simulink model "chap03"  (R2021a)
settings: Solver=FixedStepDiscrete  StartTime=0.0  StopTime=7.5  FixedStep=0.001  RelTol=1e-3
undefined symbols (not defined in the file): DiscIntNeverNeededParam
(part 1 of 3)
settings Model: Creator=陈天兴  LastModifiedBy=陈天兴

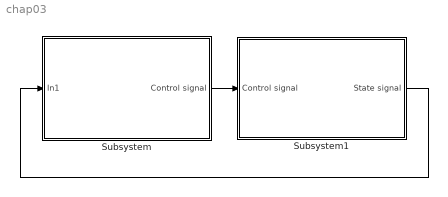
== system chap03 ==
  Subsystem : Subsystem
  Subsystem1 : Subsystem
  wires:
  Subsystem1/1(State signal) -> Subsystem/1(In1)
  Subsystem/1(Control signal) -> Subsystem1/1(Control signal)

== system chap03/Subsystem ==
  In1 : Inport
  Bus Creator : BusCreator  Inputs=6
  Bus Creator1 : BusCreator  Inputs=6
  Bus Creator2 : BusCreator  Inputs=2
  Subsystem : Subsystem
  Subsystem1 : Subsystem
  Subsystem10 : Subsystem
  Subsystem11 : Subsystem
  Subsystem12 : Subsystem
  Subsystem2 : Subsystem
  Subsystem3 : Subsystem
  Subsystem4 : Subsystem
  Subsystem5 : Subsystem
  Subsystem6 : Subsystem
  Subsystem8 : Subsystem
  Subsystem9 : Subsystem
  Control signal : Outport
  wires:
  Bus Creator2/1 -> Subsystem11/1(In19), Subsystem8/1(In19), Subsystem10/1(In19), Subsystem12/1(In19), Subsystem9/1(In19), Subsystem6/1(In19), Subsystem/1(In19), Subsystem2/1(In19), Subsystem5/1(In19), Subsystem4/1(In19), Subsystem1/1(In19), Subsystem3/1(In19)
  Subsystem5/1(u3) -> Bus Creator/3
  Subsystem3/1(u4) -> Bus Creator/4
  Subsystem1/1(u5) -> Bus Creator/5
  Subsystem/1(u1) -> Bus Creator/1
  Subsystem2/1(u2) -> Bus Creator/2
  Subsystem4/1(u6) -> Bus Creator/6
  Bus Creator/1 -> Control signal/1
  Subsystem10/1(u4) -> Bus Creator1/4
  In1/1 -> Bus Creator2/2  "state(t)"
  Bus Creator1/1 -> Bus Creator2/1  "state(tk)"
  Subsystem6/1(u1) -> Bus Creator1/1
  Subsystem9/1(u2) -> Bus Creator1/2
  Subsystem12/1(u3) -> Bus Creator1/3
  Subsystem8/1(u5) -> Bus Creator1/5
  Subsystem11/1(u6) -> Bus Creator1/6

== system chap03/Subsystem1 ==
  Control signal : Inport
  Bus Creator : BusCreator  Inputs=6
  Bus Selector : BusSelector  OutputSignals=node1.ux,node1.uy,node1.uz
  Bus Selector1 : BusSelector  OutputSignals=node2.ux,node2.uy,node2.uz
  Bus Selector2 : BusSelector  OutputSignals=node3.ux,node3.uy,node3.uz
  Bus Selector3 : BusSelector  OutputSignals=node4.ux,node4.uy,node4.uz
  Bus Selector4 : BusSelector  OutputSignals=node5.ux,node5.uy,node5.uz
  Bus Selector5 : BusSelector  OutputSignals=node6.ux,node6.uy,node6.uz
  Subsystem : Subsystem
  Subsystem1 : Subsystem
  Subsystem2 : Subsystem
  Subsystem3 : Subsystem
  Subsystem4 : Subsystem
  Subsystem5 : Subsystem
  State signal : Outport
  wires:
  Bus Creator/1 -> State signal/1
  Subsystem/1(node1) -> Bus Creator/1
  Subsystem1/1(node2) -> Bus Creator/2
  Subsystem2/1(node3) -> Bus Creator/3
  Subsystem3/1(node4) -> Bus Creator/4
  Subsystem4/1(node5) -> Bus Creator/5
  Subsystem5/1(node6) -> Bus Creator/6
  Control signal/1 -> Bus Selector2/1, Bus Selector1/1, Bus Selector/1, Bus Selector5/1, Bus Selector4/1, Bus Selector3/1
  Bus Selector/1 -> Subsystem/1(ut1x)  "<ux>"
  Bus Selector/2 -> Subsystem/2(ut1y)  "<uy>"
  Bus Selector/3 -> Subsystem/3(ut1z)  "<uz>"
  Bus Selector1/1 -> Subsystem1/1(ut2x)  "<ux>"
  Bus Selector1/2 -> Subsystem1/2(ut2y)  "<uy>"
  Bus Selector1/3 -> Subsystem1/3(ut2z)  "<uz>"
  Bus Selector2/1 -> Subsystem2/1(ut3x)  "<ux>"
  Bus Selector2/2 -> Subsystem2/2(ut3y)  "<uy>"
  Bus Selector2/3 -> Subsystem2/3(ut3z)  "<uz>"
  Bus Selector3/1 -> Subsystem3/1(ut4x)  "<ux>"
  Bus Selector3/2 -> Subsystem3/2(ut4y)  "<uy>"
  Bus Selector3/3 -> Subsystem3/3(ut4z)  "<uz>"
  Bus Selector4/1 -> Subsystem4/1(ut5x)  "<ux>"
  Bus Selector4/2 -> Subsystem4/2(ut5y)  "<uy>"
  Bus Selector4/3 -> Subsystem4/3(ut5z)  "<uz>"
  Bus Selector5/1 -> Subsystem5/1(ut6x)  "<ux>"
  Bus Selector5/2 -> Subsystem5/2(ut6y)  "<uy>"
  Bus Selector5/3 -> Subsystem5/3(ut6z)  "<uz>"

== system chap03/Subsystem/Subsystem ==
  In19 : Inport
  Bus Creator : BusCreator  Inputs=3
  Bus Selector : BusSelector  OutputSignals=state(tk).node1.xx,state(tk).node2.xx,state(tk).node3.xx,state(tk).node6.xx,state(tk).node1.vx,state(tk).node2.vx,state(tk).node3.vx,state(tk).node6.vx
  Bus Selector1 : BusSelector  OutputSignals=state(tk).node1.xy,state(tk).node2.xy,state(tk).node3.xy,state(tk).node6.xy,state(tk).node1.vy,state(tk).node2.vy,state(tk).node3.vy,state(tk).node6.vy
  Bus Selector2 : BusSelector  OutputSignals=state(tk).node1.xz,state(tk).node2.xz,state(tk).node3.xz,state(tk).node6.xz,state(tk).node1.vz,state(tk).node2.vz,state(tk).node3.vz,state(tk).node6.vz
  Subsystem1 : Subsystem
  Subsystem2 : Subsystem
  Subsystem6 : Subsystem
  u1 : Outport
  wires:
  Subsystem2/1(utx) -> Bus Creator/3  "uz"
  Subsystem6/1(utx) -> Bus Creator/1  "ux"
  Subsystem1/1(utx) -> Bus Creator/2  "uy"
  Bus Creator/1 -> u1/1  "node1"
  In19/1 -> Bus Selector2/1, Bus Selector/1, Bus Selector1/1
  Bus Selector/1 -> Subsystem6/1(xx1)  "<xx>"
  Bus Selector/2 -> Subsystem6/2(xx2)  "<xx>"
  Bus Selector/3 -> Subsystem6/3(xx3)  "<xx>"
  Bus Selector/4 -> Subsystem6/4(xx6)  "<xx>"
  Bus Selector/5 -> Subsystem6/5(vx1)  "<vx>"
  Bus Selector/6 -> Subsystem6/6(vx2)  "<vx>"
  Bus Selector/7 -> Subsystem6/7(vx3)  "<vx>"
  Bus Selector/8 -> Subsystem6/8(vx6)  "<vx>"
  Bus Selector1/1 -> Subsystem1/1(xy1)  "<xy>"
  Bus Selector1/2 -> Subsystem1/2(xy2)  "<xy>"
  Bus Selector1/3 -> Subsystem1/3(xy3)  "<xy>"
  Bus Selector1/4 -> Subsystem1/4(xy6)  "<xy>"
  Bus Selector1/5 -> Subsystem1/5(vy1)  "<vy>"
  Bus Selector1/6 -> Subsystem1/6(vy2)  "<vy>"
  Bus Selector1/7 -> Subsystem1/7(vy3)  "<vy>"
  Bus Selector1/8 -> Subsystem1/8(vy6)  "<vy>"
  Bus Selector2/1 -> Subsystem2/1(xz1)  "<xz>"
  Bus Selector2/2 -> Subsystem2/2(xx2)  "<xz>"
  Bus Selector2/3 -> Subsystem2/3(xz3)  "<xz>"
  Bus Selector2/4 -> Subsystem2/4(xz6)  "<xz>"
  Bus Selector2/5 -> Subsystem2/5(vz1)  "<vz>"
  Bus Selector2/6 -> Subsystem2/6(vz2)  "<vz>"
  Bus Selector2/7 -> Subsystem2/7(vz3)  "<vz>"
  Bus Selector2/8 -> Subsystem2/8(vz6)  "<vz>"

== system chap03/Subsystem/Subsystem1 ==
  In19 : Inport
  Bus Creator : BusCreator  Inputs=3
  Bus Selector : BusSelector  OutputSignals=state(tk).node5.xx,state(tk).node3.xx,state(tk).node4.xx,state(tk).node5.vx,state(tk).node3.vx,state(tk).node4.vx
  Bus Selector1 : BusSelector  OutputSignals=state(tk).node5.xy,state(tk).node3.xy,state(tk).node4.xy,state(tk).node5.vy,state(tk).node3.vy,state(tk).node4.vy
  Bus Selector2 : BusSelector  OutputSignals=state(tk).node5.xz,state(tk).node3.xz,state(tk).node4.xz,state(tk).node5.vz,state(tk).node3.vz,state(tk).node4.vz
  Subsystem2 : Subsystem
  Subsystem5 : Subsystem
  Subsystem6 : Subsystem
  u5 : Outport
  wires:
  Bus Creator/1 -> u5/1  "node5"
  Subsystem5/1(uty) -> Bus Creator/2  "uy"
  Subsystem6/1(utx) -> Bus Creator/1  "ux"
  Subsystem2/1(utz) -> Bus Creator/3  "uz"
  Bus Selector1/3 -> Subsystem5/3(xy4)  "<xy>"
  Bus Selector1/2 -> Subsystem5/2(xy3)  "<xy>"
  Bus Selector1/1 -> Subsystem5/1(xy5)  "<xy>"
  Bus Selector2/2 -> Subsystem2/2(xz3)  "<xz>"
  Bus Selector2/6 -> Subsystem2/6(vz4)  "<vz>"
  Bus Selector2/5 -> Subsystem2/5(vz3)  "<vz>"
  Bus Selector/4 -> Subsystem6/4(vx5)  "<vx>"
  Bus Selector1/6 -> Subsystem5/6(vy4)  "<vy>"
  Bus Selector1/4 -> Subsystem5/4(vy5)  "<vy>"
  In19/1 -> Bus Selector2/1, Bus Selector/1, Bus Selector1/1
  Bus Selector/1 -> Subsystem6/1(xx5)  "<xx>"
  Bus Selector/2 -> Subsystem6/2(xx3)  "<xx>"
  Bus Selector1/5 -> Subsystem5/5(vy3)  "<vy>"
  Bus Selector/6 -> Subsystem6/6(vx4)  "<vx>"
  Bus Selector/5 -> Subsystem6/5(vx3)  "<vx>"
  Bus Selector/3 -> Subsystem6/3(xx4)  "<xx>"
  Bus Selector2/1 -> Subsystem2/1(xz5)  "<xz>"
  Bus Selector2/3 -> Subsystem2/3(xz4)  "<xz>"
  Bus Selector2/4 -> Subsystem2/4(vz5)  "<vz>"

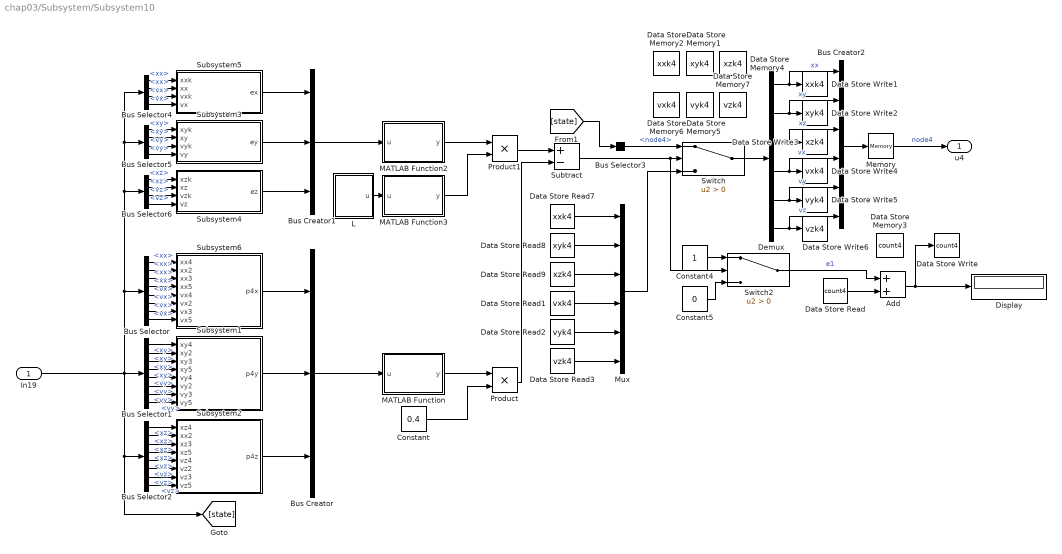
== system chap03/Subsystem/Subsystem10 ==
  In19 : Inport
  Add : Sum
  Bus Creator : BusCreator  Inputs=3
  Bus Creator1 : BusCreator  Inputs=3
  Bus Creator2 : BusCreator  Inputs=6
  Bus Selector : BusSelector  OutputSignals=state(tk).node4.xx,state(tk).node2.xx,state(tk).node3.xx,state(tk).node5.xx,state(tk).node4.vx,state(tk).node2.vx,state(tk).node3.vx,state(tk).node5.vx
  Bus Selector1 : BusSelector  OutputSignals=state(tk).node4.xy,state(tk).node2.xy,state(tk).node3.xy,state(tk).node5.xy,state(tk).node4.vy,state(tk).node2.vy,state(tk).node3.vy,state(tk).node5.vy
  Bus Selector2 : BusSelector  OutputSignals=state(tk).node4.xz,state(tk).node2.xz,state(tk).node3.xz,state(tk).node5.xz,state(tk).node4.vz,state(tk).node2.vz,state(tk).node3.vz,state(tk).node5.vz
  Bus Selector3 : BusSelector  OutputSignals=state(t).node4
  Bus Selector4 : BusSelector  OutputSignals=state(tk).node4.xx,state(t).node4.xx,state(tk).node4.vx,state(t).node4.vx
  Bus Selector5 : BusSelector  OutputSignals=state(tk).node4.xy,state(t).node4.xy,state(tk).node4.vy,state(t).node4.vy
  Bus Selector6 : BusSelector  OutputSignals=state(tk).node4.xz,state(t).node4.xz,state(tk).node4.vz,state(t).node4.vz
  Constant : Constant  Value=0.4
  Constant4 : Constant
  Constant5 : Constant  Value=0
  Data Store Memory1 : DataStoreMemory  DataStoreName=xyk4  ReadBeforeWriteMsg=warning  WriteAfterWriteMsg=warning  WriteAfterReadMsg=warning  ShowAdditionalParam=off
  Data Store Memory2 : DataStoreMemory  DataStoreName=xxk4  ReadBeforeWriteMsg=warning  WriteAfterWriteMsg=warning  WriteAfterReadMsg=warning  ShowAdditionalParam=off
  Data Store Memory3 : DataStoreMemory  DataStoreName=count4  ReadBeforeWriteMsg=warning  WriteAfterWriteMsg=warning  WriteAfterReadMsg=warning  ShowAdditionalParam=off
  Data Store Memory4 : DataStoreMemory  DataStoreName=xzk4  ReadBeforeWriteMsg=warning  WriteAfterWriteMsg=warning  WriteAfterReadMsg=warning  ShowAdditionalParam=off
  Data Store Memory5 : DataStoreMemory  DataStoreName=vyk4  ReadBeforeWriteMsg=warning  WriteAfterWriteMsg=warning  WriteAfterReadMsg=warning  ShowAdditionalParam=off
  Data Store Memory6 : DataStoreMemory  DataStoreName=vxk4  ReadBeforeWriteMsg=warning  WriteAfterWriteMsg=warning  WriteAfterReadMsg=warning  ShowAdditionalParam=off
  Data Store Memory7 : DataStoreMemory  DataStoreName=vzk4  ReadBeforeWriteMsg=warning  WriteAfterWriteMsg=warning  WriteAfterReadMsg=warning  ShowAdditionalParam=off
  Data Store Read : DataStoreRead  DataStoreName=count4  IndexOptions=Index vector (dialog)  Indices=1  OutputSizes=1
  Data Store Read1 : DataStoreRead  DataStoreName=vxk4  IndexOptions=Index vector (dialog)  Indices=1  OutputSizes=1
  Data Store Read2 : DataStoreRead  DataStoreName=vyk4  IndexOptions=Index vector (dialog)  Indices=1  OutputSizes=1
  Data Store Read3 : DataStoreRead  DataStoreName=vzk4  IndexOptions=Index vector (dialog)  Indices=1  OutputSizes=1
  Data Store Read7 : DataStoreRead  DataStoreName=xxk4  IndexOptions=Index vector (dialog)  Indices=1  OutputSizes=1
  Data Store Read8 : DataStoreRead  DataStoreName=xyk4  IndexOptions=Index vector (dialog)  Indices=1  OutputSizes=1
  Data Store Read9 : DataStoreRead  DataStoreName=xzk4  IndexOptions=Index vector (dialog)  Indices=1  OutputSizes=1
  Data Store Write : DataStoreWrite  DataStoreName=count4  IndexOptions=Index vector (dialog)  Indices=1  OutputSizes=1
  Data Store Write1 : DataStoreWrite  DataStoreName=xxk4  IndexOptions=Index vector (dialog)  Indices=1  OutputSizes=1
  Data Store Write2 : DataStoreWrite  DataStoreName=xyk4  IndexOptions=Index vector (dialog)  Indices=1  OutputSizes=1
  Data Store Write3 : DataStoreWrite  DataStoreName=xzk4  IndexOptions=Index vector (dialog)  Indices=1  OutputSizes=1
  Data Store Write4 : DataStoreWrite  DataStoreName=vxk4  IndexOptions=Index vector (dialog)  Indices=1  OutputSizes=1
  Data Store Write5 : DataStoreWrite  DataStoreName=vyk4  IndexOptions=Index vector (dialog)  Indices=1  OutputSizes=1
  Data Store Write6 : DataStoreWrite  DataStoreName=vzk4  IndexOptions=Index vector (dialog)  Indices=1  OutputSizes=1
  Demux : Demux  Outputs=6
  Display : Display
  L : Subsystem
  MATLAB Function : MATLAB Function  TreatAsAtomicUnit=on
  MATLAB Function2 : MATLAB Function  TreatAsAtomicUnit=on
  MATLAB Function3 : MATLAB Function  TreatAsAtomicUnit=on
  Memory : Memory
  Mux : Mux  Inputs=6
  Product : Product
  Product1 : Product
  Subsystem1 : Subsystem
  Subsystem2 : Subsystem
  Subsystem3 : Subsystem
  Subsystem4 : Subsystem
  Subsystem5 : Subsystem
  Subsystem6 : Subsystem
  Subtract : Sum  Inputs=+-
  Switch : Switch  Criteria=u2 > Threshold
  Switch2 : Switch  Criteria=u2 > Threshold
  u4 : Outport
  wires:
  Subsystem2/1(p4z) -> Bus Creator/3
  Subsystem6/1(p4x) -> Bus Creator/1
  Subsystem1/1(p4y) -> Bus Creator/2
  Bus Selector/1 -> Subsystem6/1(xx4)  "<xx>"
  Bus Selector/2 -> Subsystem6/2(xx2)  "<xx>"
  Bus Selector/3 -> Subsystem6/3(xx3)  "<xx>"
  Bus Selector/4 -> Subsystem6/4(xx5)  "<xx>"
  Bus Selector/5 -> Subsystem6/5(vx4)  "<vx>"
  Bus Selector/6 -> Subsystem6/6(vx2)  "<vx>"
  Bus Selector/7 -> Subsystem6/7(vx3)  "<vx>"
  Bus Selector/8 -> Subsystem6/8(vx5)  "<vx>"
  Bus Selector1/1 -> Subsystem1/1(xy4)  "<xy>"
  Bus Selector1/2 -> Subsystem1/2(xy2)  "<xy>"
  Bus Selector1/3 -> Subsystem1/3(xy3)  "<xy>"
  Bus Selector1/4 -> Subsystem1/4(xy5)  "<xy>"
  Bus Selector1/5 -> Subsystem1/5(vy4)  "<vy>"
  Bus Selector1/6 -> Subsystem1/6(vy2)  "<vy>"
  Bus Selector1/7 -> Subsystem1/7(vy3)  "<vy>"
  Bus Selector1/8 -> Subsystem1/8(vy5)  "<vy>"
  Bus Selector2/1 -> Subsystem2/1(xz4)  "<xz>"
  Bus Selector2/2 -> Subsystem2/2(xx2)  "<xz>"
  Bus Selector2/3 -> Subsystem2/3(xz3)  "<xz>"
  Bus Selector2/4 -> Subsystem2/4(xz5)  "<xz>"
  Bus Selector2/5 -> Subsystem2/5(vz4)  "<vz>"
  Bus Selector2/6 -> Subsystem2/6(vz2)  "<vz>"
  Bus Selector2/7 -> Subsystem2/7(vz3)  "<vz>"
  Bus Selector2/8 -> Subsystem2/8(vz5)  "<vz>"
  Data Store Read3/1 -> Mux/6
  Switch/1 -> Demux/1
  Demux/2 -> Bus Creator2/2, Data Store Write2/1  "xy"
  Bus Selector3/1 -> Switch/1  "<node4>"
  Demux/1 -> Bus Creator2/1, Data Store Write1/1  "xx"
  Switch2/1 -> Add/1  "e1"
  Demux/6 -> Bus Creator2/6, Data Store Write6/1  "vz"
  Demux/3 -> Bus Creator2/3, Data Store Write3/1  "xz"
  Data Store Read7/1 -> Mux/1
  Constant4/1 -> Switch2/1
  Mux/1 -> Switch/3
  Data Store Read9/1 -> Mux/3
  Add/1 -> Data Store Write/1, Display/1
  Demux/4 -> Bus Creator2/4, Data Store Write4/1  "vx"
  Bus Creator2/1 -> Memory/1
  Data Store Read2/1 -> Mux/5
  Data Store Read1/1 -> Mux/4
  Product/1 -> Subtract/2
  Data Store Read8/1 -> Mux/2
  [state] -> Bus Selector3/1
  MATLAB Function3/1(y) -> Product1/2
  Bus Creator1/1 -> MATLAB Function2/1(u)
  Constant5/1 -> Switch2/3
  Constant/1 -> Product/2
  MATLAB Function2/1(y) -> Product1/1
  Subsystem4/1(ez) -> Bus Creator1/3
  Subsystem5/1(ex) -> Bus Creator1/1
  Subsystem3/1(ey) -> Bus Creator1/2
  Demux/5 -> Bus Creator2/5, Data Store Write5/1  "vy"
  Product1/1 -> Subtract/1
  Data Store Read/1 -> Add/2
  MATLAB Function/1(y) -> Product/1
  Bus Creator/1 -> MATLAB Function/1(u)
  Bus Selector5/3 -> Subsystem3/3(vyk)  "<vy>"
  In19/1 -> [state], Bus Selector2/1, Bus Selector1/1, Bus Selector/1, Bus Selector6/1, Bus Selector5/1, Bus Selector4/1
  Bus Selector5/2 -> Subsystem3/2(xy)  "<xy>"
  Bus Selector5/4 -> Subsystem3/4(vy)  "<vy>"
  Bus Selector5/1 -> Subsystem3/1(xyk)  "<xy>"
  Bus Selector6/2 -> Subsystem4/2(xz)  "<xz>"
  Bus Selector6/3 -> Subsystem4/3(vzk)  "<vz>"
  Bus Selector6/4 -> Subsystem4/4(vz)  "<vz>"
  Bus Selector6/1 -> Subsystem4/1(xzk)  "<xz>"
  Memory/1 -> u4/1  "node4"
  Bus Selector4/1 -> Subsystem5/1(xxk)  "<xx>"
  Bus Selector4/2 -> Subsystem5/2(xx)  "<xx>"
  Bus Selector4/3 -> Subsystem5/3(vxk)  "<vx>"
  Bus Selector4/4 -> Subsystem5/4(vx)  "<vx>"
  Subtract/1 -> Switch/2, Switch2/2
  L/1(u) -> MATLAB Function3/1(u)

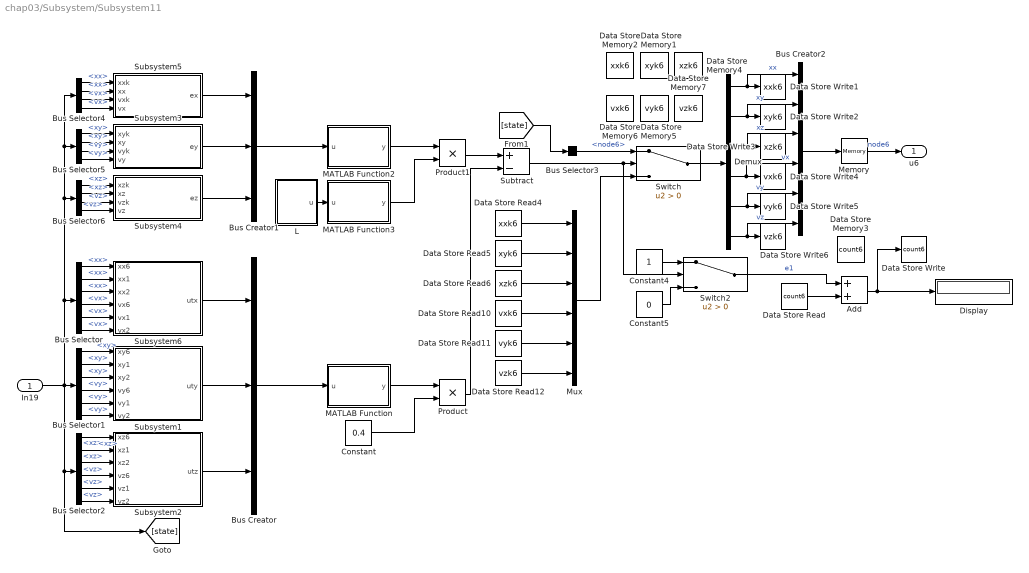
== system chap03/Subsystem/Subsystem11 ==
  In19 : Inport
  Add : Sum
  Bus Creator : BusCreator  Inputs=3
  Bus Creator1 : BusCreator  Inputs=3
  Bus Creator2 : BusCreator  Inputs=6
  Bus Selector : BusSelector  OutputSignals=state(tk).node6.xx,state(tk).node1.xx,state(tk).node2.xx,state(tk).node6.vx,state(tk).node1.vx,state(tk).node2.vx
  Bus Selector1 : BusSelector  OutputSignals=state(tk).node6.xy,state(tk).node1.xy,state(tk).node2.xy,state(tk).node6.vy,state(tk).node1.vy,state(tk).node2.vy
  Bus Selector2 : BusSelector  OutputSignals=state(tk).node6.xz,state(tk).node1.xz,state(tk).node2.xz,state(tk).node6.vz,state(tk).node1.vz,state(tk).node2.vz
  Bus Selector3 : BusSelector  OutputSignals=state(t).node6
  Bus Selector4 : BusSelector  OutputSignals=state(tk).node6.xx,state(t).node6.xx,state(tk).node6.vx,state(t).node6.vx
  Bus Selector5 : BusSelector  OutputSignals=state(tk).node6.xy,state(t).node6.xy,state(tk).node6.vy,state(t).node6.vy
  Bus Selector6 : BusSelector  OutputSignals=state(tk).node6.xz,state(t).node6.xz,state(tk).node6.vz,state(t).node6.vz
  Constant : Constant  Value=0.4
  Constant4 : Constant
  Constant5 : Constant  Value=0
  Data Store Memory1 : DataStoreMemory  DataStoreName=xyk6  ReadBeforeWriteMsg=warning  WriteAfterWriteMsg=warning  WriteAfterReadMsg=warning  ShowAdditionalParam=off
  Data Store Memory2 : DataStoreMemory  DataStoreName=xxk6  ReadBeforeWriteMsg=warning  WriteAfterWriteMsg=warning  WriteAfterReadMsg=warning  ShowAdditionalParam=off
  Data Store Memory3 : DataStoreMemory  DataStoreName=count6  ReadBeforeWriteMsg=warning  WriteAfterWriteMsg=warning  WriteAfterReadMsg=warning  ShowAdditionalParam=off
  Data Store Memory4 : DataStoreMemory  DataStoreName=xzk6  ReadBeforeWriteMsg=warning  WriteAfterWriteMsg=warning  WriteAfterReadMsg=warning  ShowAdditionalParam=off
  Data Store Memory5 : DataStoreMemory  DataStoreName=vyk6  ReadBeforeWriteMsg=warning  WriteAfterWriteMsg=warning  WriteAfterReadMsg=warning  ShowAdditionalParam=off
  Data Store Memory6 : DataStoreMemory  DataStoreName=vxk6  ReadBeforeWriteMsg=warning  WriteAfterWriteMsg=warning  WriteAfterReadMsg=warning  ShowAdditionalParam=off
  Data Store Memory7 : DataStoreMemory  DataStoreName=vzk6  ReadBeforeWriteMsg=warning  WriteAfterWriteMsg=warning  WriteAfterReadMsg=warning  ShowAdditionalParam=off
  Data Store Read : DataStoreRead  DataStoreName=count6  IndexOptions=Index vector (dialog)  Indices=1  OutputSizes=1
  Data Store Read10 : DataStoreRead  DataStoreName=vxk6  IndexOptions=Index vector (dialog)  Indices=1  OutputSizes=1
  Data Store Read11 : DataStoreRead  DataStoreName=vyk6  IndexOptions=Index vector (dialog)  Indices=1  OutputSizes=1
  Data Store Read12 : DataStoreRead  DataStoreName=vzk6  IndexOptions=Index vector (dialog)  Indices=1  OutputSizes=1
  Data Store Read4 : DataStoreRead  DataStoreName=xxk6  IndexOptions=Index vector (dialog)  Indices=1  OutputSizes=1
  Data Store Read5 : DataStoreRead  DataStoreName=xyk6  IndexOptions=Index vector (dialog)  Indices=1  OutputSizes=1
  Data Store Read6 : DataStoreRead  DataStoreName=xzk6  IndexOptions=Index vector (dialog)  Indices=1  OutputSizes=1
  Data Store Write : DataStoreWrite  DataStoreName=count6  IndexOptions=Index vector (dialog)  Indices=1  OutputSizes=1
  Data Store Write1 : DataStoreWrite  DataStoreName=xxk6  IndexOptions=Index vector (dialog)  Indices=1  OutputSizes=1
  Data Store Write2 : DataStoreWrite  DataStoreName=xyk6  IndexOptions=Index vector (dialog)  Indices=1  OutputSizes=1
  Data Store Write3 : DataStoreWrite  DataStoreName=xzk6  IndexOptions=Index vector (dialog)  Indices=1  OutputSizes=1
  Data Store Write4 : DataStoreWrite  DataStoreName=vxk6  IndexOptions=Index vector (dialog)  Indices=1  OutputSizes=1
  Data Store Write5 : DataStoreWrite  DataStoreName=vyk6  IndexOptions=Index vector (dialog)  Indices=1  OutputSizes=1
  Data Store Write6 : DataStoreWrite  DataStoreName=vzk6  IndexOptions=Index vector (dialog)  Indices=1  OutputSizes=1
  Demux : Demux  Outputs=6
  Display : Display
  L : Subsystem
  MATLAB Function : MATLAB Function  TreatAsAtomicUnit=on
  MATLAB Function2 : MATLAB Function  TreatAsAtomicUnit=on
  MATLAB Function3 : MATLAB Function  TreatAsAtomicUnit=on
  Memory : Memory
  Mux : Mux  Inputs=6
  Product : Product
  Product1 : Product
  Subsystem1 : Subsystem
  Subsystem2 : Subsystem
  Subsystem3 : Subsystem
  Subsystem4 : Subsystem
  Subsystem5 : Subsystem
  Subsystem6 : Subsystem
  Subtract : Sum  Inputs=+-
  Switch : Switch  Criteria=u2 > Threshold
  Switch2 : Switch  Criteria=u2 > Threshold
  u6 : Outport
  wires:
  Bus Selector2/6 -> Subsystem2/6(vz2)  "<vz>"
  Bus Selector2/5 -> Subsystem2/5(vz1)  "<vz>"
  Bus Selector2/4 -> Subsystem2/4(vz6)  "<vz>"
  Bus Selector2/3 -> Subsystem2/3(xz2)  "<xz>"
  Bus Selector2/1 -> Subsystem2/1(xz6)  "<xz>"
  Bus Selector2/2 -> Subsystem2/2(xz1)  "<xz>"
  Bus Selector1/6 -> Subsystem1/6(vy2)  "<vy>"
  Bus Selector1/5 -> Subsystem1/5(vy1)  "<vy>"
  Bus Selector1/4 -> Subsystem1/4(vy6)  "<vy>"
  Bus Selector1/3 -> Subsystem1/3(xy2)  "<xy>"
  Bus Selector1/2 -> Subsystem1/2(xy1)  "<xy>"
  Bus Selector1/1 -> Subsystem1/1(xy6)  "<xy>"
  Bus Selector/6 -> Subsystem6/6(vx2)  "<vx>"
  Bus Selector/5 -> Subsystem6/5(vx1)  "<vx>"
  Bus Selector/4 -> Subsystem6/4(vx6)  "<vx>"
  Bus Selector/3 -> Subsystem6/3(xx2)  "<xx>"
  Bus Selector/2 -> Subsystem6/2(xx1)  "<xx>"
  Bus Selector/1 -> Subsystem6/1(xx6)  "<xx>"
  Subsystem1/1(uty) -> Bus Creator/2
  Subsystem6/1(utx) -> Bus Creator/1
  Subsystem2/1(utz) -> Bus Creator/3
  Data Store Read/1 -> Add/2
  Subsystem3/1(ey) -> Bus Creator1/2
  Demux/4 -> Bus Creator2/4, Data Store Write4/1  "vx"
  MATLAB Function/1(y) -> Product/1
  Bus Creator/1 -> MATLAB Function/1(u)
  Product1/1 -> Subtract/1
  Data Store Read4/1 -> Mux/1
  Demux/1 -> Bus Creator2/1, Data Store Write1/1  "xx"
  Add/1 -> Data Store Write/1, Display/1
  Demux/6 -> Bus Creator2/6, Data Store Write6/1  "vz"
  Subsystem5/1(ex) -> Bus Creator1/1
  Data Store Read5/1 -> Mux/2
  Demux/5 -> Bus Creator2/5, Data Store Write5/1  "vy"
  Data Store Read11/1 -> Mux/5
  Demux/3 -> Bus Creator2/3, Data Store Write3/1  "xz"
  Subsystem4/1(ez) -> Bus Creator1/3
  Bus Creator1/1 -> MATLAB Function2/1(u)
  Data Store Read6/1 -> Mux/3
  MATLAB Function2/1(y) -> Product1/1
  Constant4/1 -> Switch2/1
  Mux/1 -> Switch/3
  Switch/1 -> Demux/1
  Constant/1 -> Product/2
  Constant5/1 -> Switch2/3
  MATLAB Function3/1(y) -> Product1/2
  Data Store Read10/1 -> Mux/4
  Data Store Read12/1 -> Mux/6
  Switch2/1 -> Add/1  "e1"
  Demux/2 -> Bus Creator2/2, Data Store Write2/1  "xy"
  Product/1 -> Subtract/2
  Memory/1 -> u6/1  "node6"
  Bus Selector3/1 -> Switch/1  "<node6>"
  [state] -> Bus Selector3/1
  Bus Selector4/4 -> Subsystem5/4(vx)  "<vx>"
  Bus Selector5/3 -> Subsystem3/3(vyk)  "<vy>"
  Bus Selector5/2 -> Subsystem3/2(xy)  "<xy>"
  Bus Selector4/1 -> Subsystem5/1(xxk)  "<xx>"
  Bus Selector5/4 -> Subsystem3/4(vy)  "<vy>"
  Bus Selector5/1 -> Subsystem3/1(xyk)  "<xy>"
  In19/1 -> Bus Selector5/1, Bus Selector4/1, Bus Selector6/1, Bus Selector/1, Bus Selector1/1, [state], Bus Selector2/1
  Bus Selector4/3 -> Subsystem5/3(vxk)  "<vx>"
  Bus Selector6/2 -> Subsystem4/2(xz)  "<xz>"
  Bus Selector6/3 -> Subsystem4/3(vzk)  "<vz>"
  Bus Selector4/2 -> Subsystem5/2(xx)  "<xx>"
  Bus Selector6/4 -> Subsystem4/4(vz)  "<vz>"
  Bus Selector6/1 -> Subsystem4/1(xzk)  "<xz>"
  Bus Creator2/1 -> Memory/1
  Subtract/1 -> Switch/2, Switch2/2
  L/1(u) -> MATLAB Function3/1(u)

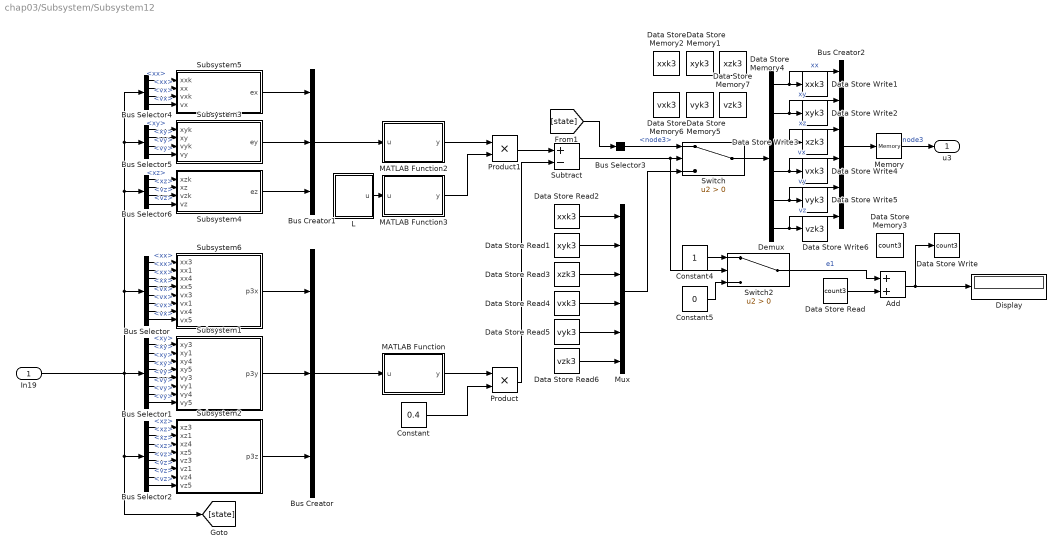
== system chap03/Subsystem/Subsystem12 ==
  In19 : Inport
  Add : Sum
  Bus Creator : BusCreator  Inputs=3
  Bus Creator1 : BusCreator  Inputs=3
  Bus Creator2 : BusCreator  Inputs=6
  Bus Selector : BusSelector  OutputSignals=state(tk).node3.xx,state(tk).node1.xx,state(tk).node4.xx,state(tk).node5.xx,state(tk).node3.vx,state(tk).node1.vx,state(tk).node4.vx,state(tk).node5.vx
  Bus Selector1 : BusSelector  OutputSignals=state(tk).node3.xy,state(tk).node1.xy,state(tk).node4.xy,state(tk).node5.xy,state(tk).node3.vy,state(tk).node1.vy,state(tk).node4.vy,state(tk).node5.vy
  Bus Selector2 : BusSelector  OutputSignals=state(tk).node3.xz,state(tk).node1.xz,state(tk).node4.xz,state(tk).node5.xz,state(tk).node3.vz,state(tk).node1.vz,state(tk).node4.vz,state(tk).node5.vz
  Bus Selector3 : BusSelector  OutputSignals=state(t).node3
  Bus Selector4 : BusSelector  OutputSignals=state(tk).node3.xx,state(t).node3.xx,state(tk).node3.vx,state(t).node3.vx
  Bus Selector5 : BusSelector  OutputSignals=state(tk).node3.xy,state(t).node3.xy,state(tk).node3.vy,state(t).node3.vy
  Bus Selector6 : BusSelector  OutputSignals=state(tk).node3.xz,state(t).node3.xz,state(tk).node3.vz,state(t).node3.vz
  Constant : Constant  Value=0.4
  Constant4 : Constant
  Constant5 : Constant  Value=0
  Data Store Memory1 : DataStoreMemory  DataStoreName=xyk3  ReadBeforeWriteMsg=warning  WriteAfterWriteMsg=warning  WriteAfterReadMsg=warning  ShowAdditionalParam=off
  Data Store Memory2 : DataStoreMemory  DataStoreName=xxk3  ReadBeforeWriteMsg=warning  WriteAfterWriteMsg=warning  WriteAfterReadMsg=warning  ShowAdditionalParam=off
  Data Store Memory3 : DataStoreMemory  DataStoreName=count3  ReadBeforeWriteMsg=warning  WriteAfterWriteMsg=warning  WriteAfterReadMsg=warning  ShowAdditionalParam=off
  Data Store Memory4 : DataStoreMemory  DataStoreName=xzk3  ReadBeforeWriteMsg=warning  WriteAfterWriteMsg=warning  WriteAfterReadMsg=warning  ShowAdditionalParam=off
  Data Store Memory5 : DataStoreMemory  DataStoreName=vyk3  ReadBeforeWriteMsg=warning  WriteAfterWriteMsg=warning  WriteAfterReadMsg=warning  ShowAdditionalParam=off
  Data Store Memory6 : DataStoreMemory  DataStoreName=vxk3  ReadBeforeWriteMsg=warning  WriteAfterWriteMsg=warning  WriteAfterReadMsg=warning  ShowAdditionalParam=off
  Data Store Memory7 : DataStoreMemory  DataStoreName=vzk3  ReadBeforeWriteMsg=warning  WriteAfterWriteMsg=warning  WriteAfterReadMsg=warning  ShowAdditionalParam=off
  Data Store Read : DataStoreRead  DataStoreName=count3  IndexOptions=Index vector (dialog)  Indices=1  OutputSizes=1
  Data Store Read1 : DataStoreRead  DataStoreName=xyk3  IndexOptions=Index vector (dialog)  Indices=1  OutputSizes=1
  Data Store Read2 : DataStoreRead  DataStoreName=xxk3  IndexOptions=Index vector (dialog)  Indices=1  OutputSizes=1
  Data Store Read3 : DataStoreRead  DataStoreName=xzk3  IndexOptions=Index vector (dialog)  Indices=1  OutputSizes=1
  Data Store Read4 : DataStoreRead  DataStoreName=vxk3  IndexOptions=Index vector (dialog)  Indices=1  OutputSizes=1
  Data Store Read5 : DataStoreRead  DataStoreName=vyk3  IndexOptions=Index vector (dialog)  Indices=1  OutputSizes=1
  Data Store Read6 : DataStoreRead  DataStoreName=vzk3  IndexOptions=Index vector (dialog)  Indices=1  OutputSizes=1
  Data Store Write : DataStoreWrite  DataStoreName=count3  IndexOptions=Index vector (dialog)  Indices=1  OutputSizes=1
  Data Store Write1 : DataStoreWrite  DataStoreName=xxk3  IndexOptions=Index vector (dialog)  Indices=1  OutputSizes=1
  Data Store Write2 : DataStoreWrite  DataStoreName=xyk3  IndexOptions=Index vector (dialog)  Indices=1  OutputSizes=1
  Data Store Write3 : DataStoreWrite  DataStoreName=xzk3  IndexOptions=Index vector (dialog)  Indices=1  OutputSizes=1
  Data Store Write4 : DataStoreWrite  DataStoreName=vxk3  IndexOptions=Index vector (dialog)  Indices=1  OutputSizes=1
  Data Store Write5 : DataStoreWrite  DataStoreName=vyk3  IndexOptions=Index vector (dialog)  Indices=1  OutputSizes=1
  Data Store Write6 : DataStoreWrite  DataStoreName=vzk3  IndexOptions=Index vector (dialog)  Indices=1  OutputSizes=1
  Demux : Demux  Outputs=6
  Display : Display
  L : Subsystem
  MATLAB Function : MATLAB Function  TreatAsAtomicUnit=on
  MATLAB Function2 : MATLAB Function  TreatAsAtomicUnit=on
  MATLAB Function3 : MATLAB Function  TreatAsAtomicUnit=on
  Memory : Memory
  Mux : Mux  Inputs=6
  Product : Product
  Product1 : Product
  Subsystem1 : Subsystem
  Subsystem2 : Subsystem
  Subsystem3 : Subsystem
  Subsystem4 : Subsystem
  Subsystem5 : Subsystem
  Subsystem6 : Subsystem
  Subtract : Sum  Inputs=+-
  Switch : Switch  Criteria=u2 > Threshold
  Switch2 : Switch  Criteria=u2 > Threshold
  u3 : Outport
  wires:
  Bus Selector2/8 -> Subsystem2/8(vz5)  "<vz>"
  Bus Selector2/7 -> Subsystem2/7(vz4)  "<vz>"
  Bus Selector2/6 -> Subsystem2/6(vz1)  "<vz>"
  Bus Selector2/5 -> Subsystem2/5(vz3)  "<vz>"
  Bus Selector2/4 -> Subsystem2/4(xz5)  "<xz>"
  Bus Selector2/3 -> Subsystem2/3(xz4)  "<xz>"
  Bus Selector2/2 -> Subsystem2/2(xz1)  "<xz>"
  Bus Selector2/1 -> Subsystem2/1(xz3)  "<xz>"
  Bus Selector1/8 -> Subsystem1/8(vy5)  "<vy>"
  Bus Selector1/7 -> Subsystem1/7(vy4)  "<vy>"
  Bus Selector1/6 -> Subsystem1/6(vy1)  "<vy>"
  Bus Selector1/5 -> Subsystem1/5(vy3)  "<vy>"
  Bus Selector1/4 -> Subsystem1/4(xy5)  "<xy>"
  Bus Selector1/3 -> Subsystem1/3(xy4)  "<xy>"
  Bus Selector1/2 -> Subsystem1/2(xy1)  "<xy>"
  Bus Selector1/1 -> Subsystem1/1(xy3)  "<xy>"
  Bus Selector/8 -> Subsystem6/8(vx5)  "<vx>"
  Bus Selector/7 -> Subsystem6/7(vx4)  "<vx>"
  Bus Selector/6 -> Subsystem6/6(vx1)  "<vx>"
  Bus Selector/5 -> Subsystem6/5(vx3)  "<vx>"
  Bus Selector/4 -> Subsystem6/4(xx5)  "<xx>"
  Bus Selector/3 -> Subsystem6/3(xx4)  "<xx>"
  Bus Selector/2 -> Subsystem6/2(xx1)  "<xx>"
  Bus Selector/1 -> Subsystem6/1(xx3)  "<xx>"
  Subsystem1/1(p3y) -> Bus Creator/2
  Subsystem6/1(p3x) -> Bus Creator/1
  Subsystem2/1(p3z) -> Bus Creator/3
  Data Store Read6/1 -> Mux/6
  Switch/1 -> Demux/1
  Demux/2 -> Bus Creator2/2, Data Store Write2/1  "xy"
  Bus Selector3/1 -> Switch/1  "<node3>"
  Demux/1 -> Bus Creator2/1, Data Store Write1/1  "xx"
  Switch2/1 -> Add/1  "e1"
  Demux/6 -> Bus Creator2/6, Data Store Write6/1  "vz"
  Demux/3 -> Bus Creator2/3, Data Store Write3/1  "xz"
  Data Store Read2/1 -> Mux/1
  Constant4/1 -> Switch2/1
  Mux/1 -> Switch/3
  Data Store Read3/1 -> Mux/3
  Add/1 -> Data Store Write/1, Display/1
  Demux/4 -> Bus Creator2/4, Data Store Write4/1  "vx"
  Memory/1 -> u3/1  "node3"
  Data Store Read5/1 -> Mux/5
  Data Store Read4/1 -> Mux/4
  Product/1 -> Subtract/2
  Data Store Read1/1 -> Mux/2
  [state] -> Bus Selector3/1
  MATLAB Function3/1(y) -> Product1/2
  Bus Creator1/1 -> MATLAB Function2/1(u)
  Constant5/1 -> Switch2/3
  Constant/1 -> Product/2
  MATLAB Function2/1(y) -> Product1/1
  Subsystem4/1(ez) -> Bus Creator1/3
  Subsystem5/1(ex) -> Bus Creator1/1
  Subsystem3/1(ey) -> Bus Creator1/2
  Demux/5 -> Bus Creator2/5, Data Store Write5/1  "vy"
  Product1/1 -> Subtract/1
  Data Store Read/1 -> Add/2
  MATLAB Function/1(y) -> Product/1
  Bus Creator/1 -> MATLAB Function/1(u)
  Bus Selector6/4 -> Subsystem4/4(vz)  "<vz>"
  Bus Selector6/2 -> Subsystem4/2(xz)  "<xz>"
  Bus Selector6/3 -> Subsystem4/3(vzk)  "<vz>"
  Bus Selector6/1 -> Subsystem4/1(xzk)  "<xz>"
  Bus Selector5/3 -> Subsystem3/3(vyk)  "<vy>"
  Bus Selector5/2 -> Subsystem3/2(xy)  "<xy>"
  Bus Selector5/4 -> Subsystem3/4(vy)  "<vy>"
  Bus Selector5/1 -> Subsystem3/1(xyk)  "<xy>"
  In19/1 -> [state], Bus Selector2/1, Bus Selector/1, Bus Selector6/1, Bus Selector5/1, Bus Selector4/1, Bus Selector1/1
  Bus Selector4/1 -> Subsystem5/1(xxk)  "<xx>"
  Bus Selector4/2 -> Subsystem5/2(xx)  "<xx>"
  Bus Selector4/3 -> Subsystem5/3(vxk)  "<vx>"
  Bus Selector4/4 -> Subsystem5/4(vx)  "<vx>"
  Bus Creator2/1 -> Memory/1
  Subtract/1 -> Switch2/2, Switch/2
  L/1(u) -> MATLAB Function3/1(u)

== system chap03/Subsystem/Subsystem2 ==
  In19 : Inport
  Bus Creator : BusCreator  Inputs=3
  Bus Selector : BusSelector  OutputSignals=state(tk).node2.xx,state(tk).node1.xx,state(tk).node4.xx,state(tk).node6.xx,state(tk).node2.vx,state(tk).node1.vx,state(tk).node4.vx,state(tk).node6.vx
  Bus Selector1 : BusSelector  OutputSignals=state(tk).node2.xy,state(tk).node1.xy,state(tk).node4.xy,state(tk).node6.xy,state(tk).node2.vy,state(tk).node1.vy,state(tk).node4.vy,state(tk).node6.vy
  Bus Selector2 : BusSelector  OutputSignals=state(tk).node2.xz,state(tk).node1.xz,state(tk).node4.xz,state(tk).node6.xz,state(tk).node2.vz,state(tk).node1.vz,state(tk).node4.vz,state(tk).node6.vz
  Subsystem1 : Subsystem
  Subsystem2 : Subsystem
  Subsystem6 : Subsystem
  u2 : Outport
  wires:
  Bus Creator/1 -> u2/1  "node2"
  Subsystem1/1(uty) -> Bus Creator/2  "uy"
  Subsystem6/1(utx) -> Bus Creator/1  "ux"
  Subsystem2/1(utz) -> Bus Creator/3  "uz"
  Bus Selector2/1 -> Subsystem2/1(xz2)  "<xz>"
  In19/1 -> Bus Selector2/1, Bus Selector/1, Bus Selector1/1
  Bus Selector/3 -> Subsystem6/3(xx4)  "<xx>"
  Bus Selector/5 -> Subsystem6/5(vx2)  "<vx>"
  Bus Selector/1 -> Subsystem6/1(xx2)  "<xx>"
  Bus Selector/7 -> Subsystem6/7(vx4)  "<vx>"
  Bus Selector1/2 -> Subsystem1/2(xy1)  "<xy>"
  Bus Selector2/4 -> Subsystem2/4(xz6)  "<xz>"
  Bus Selector2/6 -> Subsystem2/6(vz1)  "<vz>"
  Bus Selector1/1 -> Subsystem1/1(xy2)  "<xy>"
  Bus Selector2/7 -> Subsystem2/7(vz4)  "<vz>"
  Bus Selector2/5 -> Subsystem2/5(vz2)  "<vz>"
  Bus Selector1/6 -> Subsystem1/6(vy1)  "<vy>"
  Bus Selector/2 -> Subsystem6/2(xx1)  "<xx>"
  Bus Selector1/8 -> Subsystem1/8(vy6)  "<vy>"
  Bus Selector2/8 -> Subsystem2/8(vz6)  "<vz>"
  Bus Selector1/7 -> Subsystem1/7(vy4)  "<vy>"
  Bus Selector2/2 -> Subsystem2/2(xz1)  "<xz>"
  Bus Selector/8 -> Subsystem6/8(vx6)  "<vx>"
  Bus Selector1/3 -> Subsystem1/3(xy4)  "<xy>"
  Bus Selector/6 -> Subsystem6/6(vx1)  "<vx>"
  Bus Selector1/4 -> Subsystem1/4(xy6)  "<xy>"
  Bus Selector1/5 -> Subsystem1/5(vy2)  "<vy>"
  Bus Selector2/3 -> Subsystem2/3(xz4)  "<xz>"
  Bus Selector/4 -> Subsystem6/4(xx6)  "<xx>"

== system chap03/Subsystem/Subsystem3 ==
  In19 : Inport
  Bus Creator : BusCreator  Inputs=3
  Bus Selector : BusSelector  OutputSignals=state(tk).node4.xx,state(tk).node2.xx,state(tk).node3.xx,state(tk).node5.xx,state(tk).node4.vx,state(tk).node2.vx,state(tk).node3.vx,state(tk).node5.vx
  Bus Selector1 : BusSelector  OutputSignals=state(tk).node4.xy,state(tk).node2.xy,state(tk).node3.xy,state(tk).node5.xy,state(tk).node4.vy,state(tk).node2.vy,state(tk).node3.vy,state(tk).node5.vy
  Bus Selector2 : BusSelector  OutputSignals=state(tk).node4.xz,state(tk).node2.xz,state(tk).node3.xz,state(tk).node5.xz,state(tk).node4.vz,state(tk).node2.vz,state(tk).node3.vz,state(tk).node5.vz
  Subsystem1 : Subsystem
  Subsystem2 : Subsystem
  Subsystem6 : Subsystem
  u4 : Outport
  wires:
  Bus Creator/1 -> u4/1  "node4"
  Subsystem1/1(utx) -> Bus Creator/2  "uy"
  Subsystem6/1(utx) -> Bus Creator/1  "ux"
  Subsystem2/1(utx) -> Bus Creator/3  "uz"
  Bus Selector/2 -> Subsystem6/2(xx2)  "<xx>"
  Bus Selector1/7 -> Subsystem1/7(vy3)  "<vy>"
  Bus Selector1/4 -> Subsystem1/4(xy5)  "<xy>"
  Bus Selector2/3 -> Subsystem2/3(xz3)  "<xz>"
  Bus Selector/8 -> Subsystem6/8(vx5)  "<vx>"
  Bus Selector2/2 -> Subsystem2/2(xx2)  "<xz>"
  Bus Selector2/4 -> Subsystem2/4(xz5)  "<xz>"
  Bus Selector1/5 -> Subsystem1/5(vy4)  "<vy>"
  Bus Selector1/2 -> Subsystem1/2(xy2)  "<xy>"
  Bus Selector2/7 -> Subsystem2/7(vz3)  "<vz>"
  Bus Selector2/5 -> Subsystem2/5(vz4)  "<vz>"
  Bus Selector1/6 -> Subsystem1/6(vy2)  "<vy>"
  Bus Selector2/8 -> Subsystem2/8(vz5)  "<vz>"
  Bus Selector2/6 -> Subsystem2/6(vz2)  "<vz>"
  Bus Selector1/3 -> Subsystem1/3(xy3)  "<xy>"
  Bus Selector2/1 -> Subsystem2/1(xz4)  "<xz>"
  Bus Selector/5 -> Subsystem6/5(vx4)  "<vx>"
  Bus Selector/1 -> Subsystem6/1(xx4)  "<xx>"
  Bus Selector/3 -> Subsystem6/3(xx3)  "<xx>"
  In19/1 -> Bus Selector2/1, Bus Selector/1, Bus Selector1/1
  Bus Selector1/8 -> Subsystem1/8(vy5)  "<vy>"
  Bus Selector1/1 -> Subsystem1/1(xy4)  "<xy>"
  Bus Selector/7 -> Subsystem6/7(vx3)  "<vx>"
  Bus Selector/6 -> Subsystem6/6(vx2)  "<vx>"
  Bus Selector/4 -> Subsystem6/4(xx5)  "<xx>"

== system chap03/Subsystem/Subsystem4 ==
  In19 : Inport
  Bus Creator : BusCreator  Inputs=3
  Bus Selector : BusSelector  OutputSignals=state(tk).node6.xx,state(tk).node1.xx,state(tk).node2.xx,state(tk).node6.vx,state(tk).node1.vx,state(tk).node2.vx
  Bus Selector1 : BusSelector  OutputSignals=state(tk).node6.xy,state(tk).node1.xy,state(tk).node2.xy,state(tk).node6.vy,state(tk).node1.vy,state(tk).node2.vy
  Bus Selector2 : BusSelector  OutputSignals=state(tk).node6.xz,state(tk).node1.xz,state(tk).node2.xz,state(tk).node6.vz,state(tk).node1.vz,state(tk).node2.vz
  Subsystem1 : Subsystem
  Subsystem2 : Subsystem
  Subsystem6 : Subsystem
  u6 : Outport
  wires:
  Subsystem2/1(utz) -> Bus Creator/3  "uz"
  Subsystem6/1(utx) -> Bus Creator/1  "ux"
  Subsystem1/1(uty) -> Bus Creator/2  "uy"
  Bus Creator/1 -> u6/1  "node6"
  Bus Selector/1 -> Subsystem6/1(xx6)  "<xx>"
  Bus Selector/2 -> Subsystem6/2(xx1)  "<xx>"
  In19/1 -> Bus Selector2/1, Bus Selector/1, Bus Selector1/1
  Bus Selector2/3 -> Subsystem2/3(xz2)  "<xz>"
  Bus Selector/3 -> Subsystem6/3(xx2)  "<xx>"
  Bus Selector1/1 -> Subsystem1/1(xy6)  "<xy>"
  Bus Selector/4 -> Subsystem6/4(vx6)  "<vx>"
  Bus Selector1/2 -> Subsystem1/2(xy1)  "<xy>"
  Bus Selector/5 -> Subsystem6/5(vx1)  "<vx>"
  Bus Selector1/3 -> Subsystem1/3(xy2)  "<xy>"
  Bus Selector2/5 -> Subsystem2/5(vz1)  "<vz>"
  Bus Selector1/4 -> Subsystem1/4(vy6)  "<vy>"
  Bus Selector1/5 -> Subsystem1/5(vy1)  "<vy>"
  Bus Selector1/6 -> Subsystem1/6(vy2)  "<vy>"
  Bus Selector2/4 -> Subsystem2/4(vz6)  "<vz>"
  Bus Selector/6 -> Subsystem6/6(vx2)  "<vx>"
  Bus Selector2/2 -> Subsystem2/2(xz1)  "<xz>"
  Bus Selector2/1 -> Subsystem2/1(xz6)  "<xz>"
  Bus Selector2/6 -> Subsystem2/6(vz2)  "<vz>"

== system chap03/Subsystem/Subsystem5 ==
  In19 : Inport
  Bus Creator : BusCreator  Inputs=3
  Bus Selector : BusSelector  OutputSignals=state(tk).node3.xx,state(tk).node1.xx,state(tk).node4.xx,state(tk).node5.xx,state(tk).node3.vx,state(tk).node1.vx,state(tk).node4.vx,state(tk).node5.vx
  Bus Selector1 : BusSelector  OutputSignals=state(tk).node3.xy,state(tk).node1.xy,state(tk).node4.xy,state(tk).node5.xy,state(tk).node3.vy,state(tk).node1.vy,state(tk).node4.vy,state(tk).node5.vy
  Bus Selector2 : BusSelector  OutputSignals=state(tk).node3.xz,state(tk).node1.xz,state(tk).node4.xz,state(tk).node5.xz,state(tk).node3.vz,state(tk).node1.vz,state(tk).node4.vz,state(tk).node5.vz
  Subsystem1 : Subsystem
  Subsystem2 : Subsystem
  Subsystem6 : Subsystem
  u3 : Outport
  wires:
  Subsystem2/1(utz) -> Bus Creator/3  "uz"
  Subsystem6/1(utx) -> Bus Creator/1  "ux"
  Subsystem1/1(uty) -> Bus Creator/2  "uy"
  Bus Creator/1 -> u3/1  "node3"
  Bus Selector/7 -> Subsystem6/7(vx4)  "<vx>"
  In19/1 -> Bus Selector2/1, Bus Selector/1, Bus Selector1/1
  Bus Selector2/6 -> Subsystem2/6(vz1)  "<vz>"
  Bus Selector/8 -> Subsystem6/8(vx5)  "<vx>"
  Bus Selector1/1 -> Subsystem1/1(xy3)  "<xy>"
  Bus Selector/2 -> Subsystem6/2(xx1)  "<xx>"
  Bus Selector2/3 -> Subsystem2/3(xz4)  "<xz>"
  Bus Selector2/2 -> Subsystem2/2(xz1)  "<xz>"
  Bus Selector/5 -> Subsystem6/5(vx3)  "<vx>"
  Bus Selector/1 -> Subsystem6/1(xx3)  "<xx>"
  Bus Selector1/7 -> Subsystem1/7(vy4)  "<vy>"
  Bus Selector/3 -> Subsystem6/3(xx4)  "<xx>"
  Bus Selector/6 -> Subsystem6/6(vx1)  "<vx>"
  Bus Selector1/2 -> Subsystem1/2(xy1)  "<xy>"
  Bus Selector1/5 -> Subsystem1/5(vy3)  "<vy>"
  Bus Selector1/8 -> Subsystem1/8(vy5)  "<vy>"
  Bus Selector2/1 -> Subsystem2/1(xz3)  "<xz>"
  Bus Selector1/4 -> Subsystem1/4(xy5)  "<xy>"
  Bus Selector1/3 -> Subsystem1/3(xy4)  "<xy>"
  Bus Selector/4 -> Subsystem6/4(xx5)  "<xx>"
  Bus Selector2/5 -> Subsystem2/5(vz3)  "<vz>"
  Bus Selector2/7 -> Subsystem2/7(vz4)  "<vz>"
  Bus Selector1/6 -> Subsystem1/6(vy1)  "<vy>"
  Bus Selector2/8 -> Subsystem2/8(vz5)  "<vz>"
  Bus Selector2/4 -> Subsystem2/4(xz5)  "<xz>"

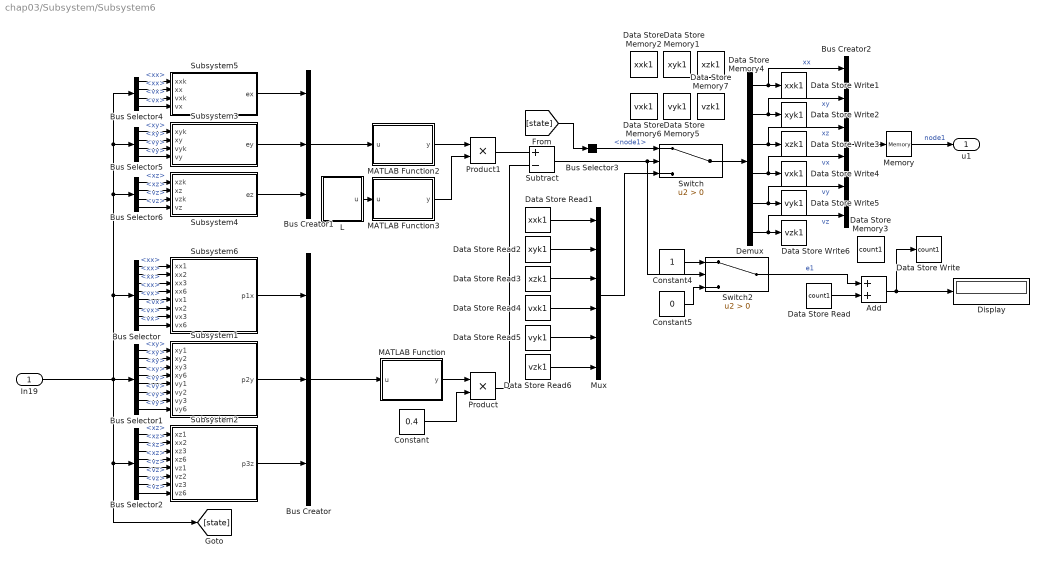
== system chap03/Subsystem/Subsystem6 ==
  In19 : Inport
  Add : Sum
  Bus Creator : BusCreator  Inputs=3
  Bus Creator1 : BusCreator  Inputs=3
  Bus Creator2 : BusCreator  Inputs=6
  Bus Selector : BusSelector  OutputSignals=state(tk).node1.xx,state(tk).node2.xx,state(tk).node3.xx,state(tk).node6.xx,state(tk).node1.vx,state(tk).node2.vx,state(tk).node3.vx,state(tk).node6.vx
  Bus Selector1 : BusSelector  OutputSignals=state(tk).node1.xy,state(tk).node2.xy,state(tk).node3.xy,state(tk).node6.xy,state(tk).node1.vy,state(tk).node2.vy,state(tk).node3.vy,state(tk).node6.vy
  Bus Selector2 : BusSelector  OutputSignals=state(tk).node1.xz,state(tk).node2.xz,state(tk).node3.xz,state(tk).node6.xz,state(tk).node1.vz,state(tk).node2.vz,state(tk).node3.vz,state(tk).node6.vz
  Bus Selector3 : BusSelector  OutputSignals=state(t).node1
  Bus Selector4 : BusSelector  OutputSignals=state(tk).node1.xx,state(t).node1.xx,state(tk).node1.vx,state(t).node1.vx
  Bus Selector5 : BusSelector  OutputSignals=state(tk).node1.xy,state(t).node1.xy,state(tk).node1.vy,state(t).node1.vy
  Bus Selector6 : BusSelector  OutputSignals=state(tk).node1.xz,state(t).node1.xz,state(tk).node1.vz,state(t).node1.vz
  Constant : Constant  Value=0.4
  Constant4 : Constant
  Constant5 : Constant  Value=0
  Data Store Memory1 : DataStoreMemory  DataStoreName=xyk1  ReadBeforeWriteMsg=warning  WriteAfterWriteMsg=warning  WriteAfterReadMsg=warning  ShowAdditionalParam=off
  Data Store Memory2 : DataStoreMemory  DataStoreName=xxk1  ReadBeforeWriteMsg=warning  WriteAfterWriteMsg=warning  WriteAfterReadMsg=warning  ShowAdditionalParam=off
  Data Store Memory3 : DataStoreMemory  DataStoreName=count1  ReadBeforeWriteMsg=warning  WriteAfterWriteMsg=warning  WriteAfterReadMsg=warning  ShowAdditionalParam=off
  Data Store Memory4 : DataStoreMemory  DataStoreName=xzk1  ReadBeforeWriteMsg=warning  WriteAfterWriteMsg=warning  WriteAfterReadMsg=warning  ShowAdditionalParam=off
  Data Store Memory5 : DataStoreMemory  DataStoreName=vyk1  ReadBeforeWriteMsg=warning  WriteAfterWriteMsg=warning  WriteAfterReadMsg=warning  ShowAdditionalParam=off
  Data Store Memory6 : DataStoreMemory  DataStoreName=vxk1  ReadBeforeWriteMsg=warning  WriteAfterWriteMsg=warning  WriteAfterReadMsg=warning  ShowAdditionalParam=off
  Data Store Memory7 : DataStoreMemory  DataStoreName=vzk1  ReadBeforeWriteMsg=warning  WriteAfterWriteMsg=warning  WriteAfterReadMsg=warning  ShowAdditionalParam=off
  Data Store Read : DataStoreRead  DataStoreName=count1  IndexOptions=Index vector (dialog)  Indices=1  OutputSizes=1
  Data Store Read1 : DataStoreRead  DataStoreName=xxk1  IndexOptions=Index vector (dialog)  Indices=1  OutputSizes=1
  Data Store Read2 : DataStoreRead  DataStoreName=xyk1  IndexOptions=Index vector (dialog)  Indices=1  OutputSizes=1
  Data Store Read3 : DataStoreRead  DataStoreName=xzk1  IndexOptions=Index vector (dialog)  Indices=1  OutputSizes=1
  Data Store Read4 : DataStoreRead  DataStoreName=vxk1  IndexOptions=Index vector (dialog)  Indices=1  OutputSizes=1
  Data Store Read5 : DataStoreRead  DataStoreName=vyk1  IndexOptions=Index vector (dialog)  Indices=1  OutputSizes=1
  Data Store Read6 : DataStoreRead  DataStoreName=vzk1  IndexOptions=Index vector (dialog)  Indices=1  OutputSizes=1
  Data Store Write : DataStoreWrite  DataStoreName=count1  IndexOptions=Index vector (dialog)  Indices=1  OutputSizes=1
  Data Store Write1 : DataStoreWrite  DataStoreName=xxk1  IndexOptions=Index vector (dialog)  Indices=1  OutputSizes=1
  Data Store Write2 : DataStoreWrite  DataStoreName=xyk1  IndexOptions=Index vector (dialog)  Indices=1  OutputSizes=1
  Data Store Write3 : DataStoreWrite  DataStoreName=xzk1  IndexOptions=Index vector (dialog)  Indices=1  OutputSizes=1
  Data Store Write4 : DataStoreWrite  DataStoreName=vxk1  IndexOptions=Index vector (dialog)  Indices=1  OutputSizes=1
  Data Store Write5 : DataStoreWrite  DataStoreName=vyk1  IndexOptions=Index vector (dialog)  Indices=1  OutputSizes=1
  Data Store Write6 : DataStoreWrite  DataStoreName=vzk1  IndexOptions=Index vector (dialog)  Indices=1  OutputSizes=1
  Demux : Demux  Outputs=6
  Display : Display
  L : Subsystem
  MATLAB Function : MATLAB Function  TreatAsAtomicUnit=on
  MATLAB Function2 : MATLAB Function  TreatAsAtomicUnit=on
  MATLAB Function3 : MATLAB Function  TreatAsAtomicUnit=on
  Memory : Memory
  Mux : Mux  Inputs=6
  Product : Product
  Product1 : Product
  Subsystem1 : Subsystem
  Subsystem2 : Subsystem
  Subsystem3 : Subsystem
  Subsystem4 : Subsystem
  Subsystem5 : Subsystem
  Subsystem6 : Subsystem
  Subtract : Sum  Inputs=+-
  Switch : Switch  Criteria=u2 > Threshold
  Switch2 : Switch  Criteria=u2 > Threshold
  u1 : Outport
  wires:
  Bus Selector2/8 -> Subsystem2/8(vz6)  "<vz>"
  Bus Selector2/7 -> Subsystem2/7(vz3)  "<vz>"
  Bus Selector2/6 -> Subsystem2/6(vz2)  "<vz>"
  Bus Selector2/5 -> Subsystem2/5(vz1)  "<vz>"
  Bus Selector2/4 -> Subsystem2/4(xz6)  "<xz>"
  Bus Selector2/3 -> Subsystem2/3(xz3)  "<xz>"
  Bus Selector2/2 -> Subsystem2/2(xx2)  "<xz>"
  Bus Selector2/1 -> Subsystem2/1(xz1)  "<xz>"
  Bus Selector1/8 -> Subsystem1/8(vy6)  "<vy>"
  Bus Selector1/7 -> Subsystem1/7(vy3)  "<vy>"
  Bus Selector1/6 -> Subsystem1/6(vy2)  "<vy>"
  Bus Selector1/5 -> Subsystem1/5(vy1)  "<vy>"
  Bus Selector1/4 -> Subsystem1/4(xy6)  "<xy>"
  Bus Selector1/3 -> Subsystem1/3(xy3)  "<xy>"
  Bus Selector1/2 -> Subsystem1/2(xy2)  "<xy>"
  Bus Selector1/1 -> Subsystem1/1(xy1)  "<xy>"
  Bus Selector/8 -> Subsystem6/8(vx6)  "<vx>"
  Bus Selector/7 -> Subsystem6/7(vx3)  "<vx>"
  Bus Selector/6 -> Subsystem6/6(vx2)  "<vx>"
  Bus Selector/5 -> Subsystem6/5(vx1)  "<vx>"
  Bus Selector/4 -> Subsystem6/4(xx6)  "<xx>"
  Bus Selector/3 -> Subsystem6/3(xx3)  "<xx>"
  Bus Selector/2 -> Subsystem6/2(xx2)  "<xx>"
  Bus Selector/1 -> Subsystem6/1(xx1)  "<xx>"
  Bus Creator/1 -> MATLAB Function/1(u)
  Subsystem1/1(p2y) -> Bus Creator/2
  Subsystem6/1(p1x) -> Bus Creator/1
  Subsystem2/1(p3z) -> Bus Creator/3
  MATLAB Function/1(y) -> Product/1
  Constant/1 -> Product/2
  Subsystem4/1(ez) -> Bus Creator1/3
  Subsystem5/1(ex) -> Bus Creator1/1
  Subsystem3/1(ey) -> Bus Creator1/2
  Bus Creator1/1 -> MATLAB Function2/1(u)
  MATLAB Function2/1(y) -> Product1/1
  L/1(u) -> MATLAB Function3/1(u)
  MATLAB Function3/1(y) -> Product1/2
  Memory/1 -> u1/1  "node1"
  Data Store Read5/1 -> Mux/5
  Data Store Read/1 -> Add/2
  Product1/1 -> Subtract/1
  Add/1 -> Display/1, Data Store Write/1
  Mux/1 -> Switch/3
  Constant4/1 -> Switch2/1
  Data Store Read3/1 -> Mux/3
  Data Store Read1/1 -> Mux/1
  Bus Selector3/1 -> Switch/1  "<node1>"
  Constant5/1 -> Switch2/3
  Switch2/1 -> Add/1  "e1"
  Data Store Read6/1 -> Mux/6
  Switch/1 -> Demux/1
  Data Store Read2/1 -> Mux/2
  Data Store Read4/1 -> Mux/4
  [state] -> Bus Selector3/1
  Demux/1 -> Bus Creator2/1, Data Store Write1/1  "xx"
  Demux/2 -> Bus Creator2/2, Data Store Write2/1  "xy"
  Demux/3 -> Bus Creator2/3, Data Store Write3/1  "xz"
  Demux/4 -> Bus Creator2/4, Data Store Write4/1  "vx"
  Demux/5 -> Bus Creator2/5, Data Store Write5/1  "vy"
  Demux/6 -> Bus Creator2/6, Data Store Write6/1  "vz"
  In19/1 -> [state], Bus Selector2/1, Bus Selector/1, Bus Selector6/1, Bus Selector5/1, Bus Selector4/1, Bus Selector1/1
  Bus Selector6/1 -> Subsystem4/1(xzk)  "<xz>"
  Bus Selector6/2 -> Subsystem4/2(xz)  "<xz>"
  Bus Selector6/3 -> Subsystem4/3(vzk)  "<vz>"
  Bus Selector6/4 -> Subsystem4/4(vz)  "<vz>"
  Bus Selector4/3 -> Subsystem5/3(vxk)  "<vx>"
  Bus Selector4/2 -> Subsystem5/2(xx)  "<xx>"
  Bus Selector4/1 -> Subsystem5/1(xxk)  "<xx>"
  Bus Selector4/4 -> Subsystem5/4(vx)  "<vx>"
  Bus Selector5/1 -> Subsystem3/1(xyk)  "<xy>"
  Bus Selector5/2 -> Subsystem3/2(xy)  "<xy>"
  Bus Selector5/3 -> Subsystem3/3(vyk)  "<vy>"
  Bus Selector5/4 -> Subsystem3/4(vy)  "<vy>"
  Bus Creator2/1 -> Memory/1
  Subtract/1 -> Switch/2, Switch2/2
  Product/1 -> Subtract/2
